simulink library "libbha_control_actuator"  (R2013b)
settings: Solver=FixedStepDiscrete  StartTime=0.0  StopTime=Inf  FixedStep=0.004  RelTol=1e-3
PostLoadFcn:
  | , if any(exist('dsrtsu_mdlpostloadfcn', 'file') == [2, 3, 6]), try dsrtsu_mdlpostloadfcn('Execute', bdroot); catch fprintf('Error in PostLoadFcn (dsrtsu_mdlpostloadfcn) for model "%s":\n %s\n', bdroot, lasterr); end, end,
undefined symbols (not defined in the file or in its folder): CONST, dim, DiscIntNeverNeededParam, tA
libraries: libbha_kinematic_tools x18, simulink x6, libbha_control_actuator x5, libbha_kinetic_cc x5, libc_control x1, libbha_parts_bellows x1, libbha_parameters x1
settings Model: DSRTSU_INTERNAL_RTI_VER=440  DSRTSU_INTERNAL_RTI_TYPE=rti1005  DSRTSU_INTERNAL_RTIFPGA=30  Creator=Falkenhahn  LastModifiedBy=Falkenhahn

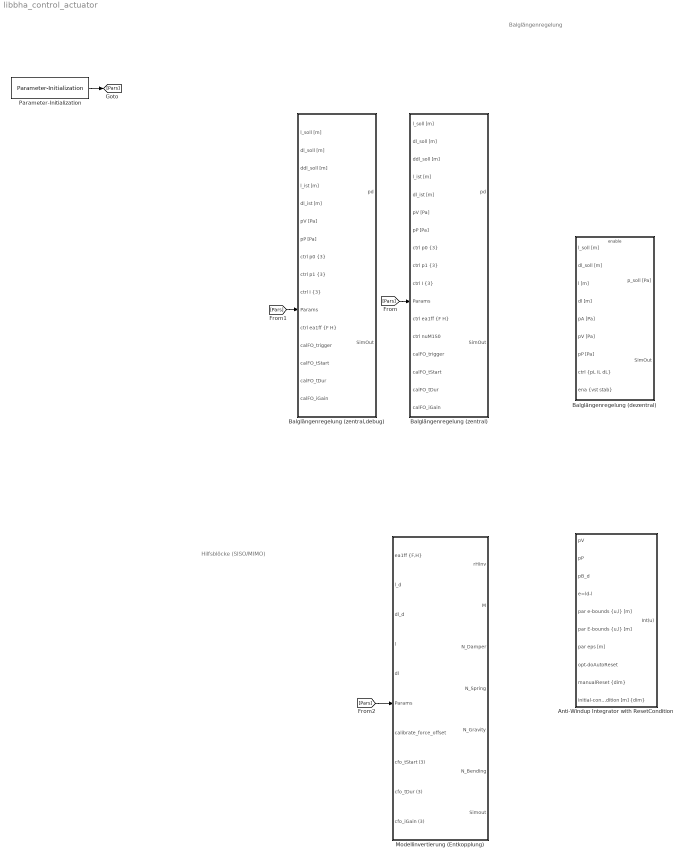
== system libbha_control_actuator ==
  note: Balglängenregelung
  note: Hilfsblöcke (SISO/MIMO)
  Anti-Windup Integrator with ResetCondition : Subsystem
      settings: AttributesFormatString=Parameter 'dim' needed\n(dimension)
  Balglängenregelung (dezentral) : Subsystem  mask{seldim=3}
      mask prompts: seldim "Dimension"
      mask init:
      | if seldim == 1
      |     dim = 1;
      | elseif seldim == 2
      |     dim = 3;
      | elseif seldim == 3
      |     dim = 6;
      | elseif seldim == 4
      |     dim = 9;
      | else
      |     dim = 1;
      | end
      settings: AttributesFormatString=%<seldim>-dimensional
      mask TypeOptions seldim: 1 | 3 | 6 | 9
  Balglängenregelung (zentral) : Subsystem
  Balglängenregelung (zentral,debug) : Subsystem
  Modellinvertierung (Entkopplung) : Subsystem
  Parameter-Initialization : libbha_parameters/Parameter-Initialization  bha_var_choice=BHA  tA=CONST.tA
      settings: AttributesFormatString=|
      | BHA-Variable: %<bha_var_choice>
      | sample time: %<tA>
  wires:
  [Pars] -> Balglängenregelung (zentral)/11(Params)
  [Pars] -> Balglängenregelung (zentral,debug)/11(Params)
  Parameter-Initialization/1 -> [Pars]
  [Pars] -> Modellinvertierung (Entkopplung)/6(Params)

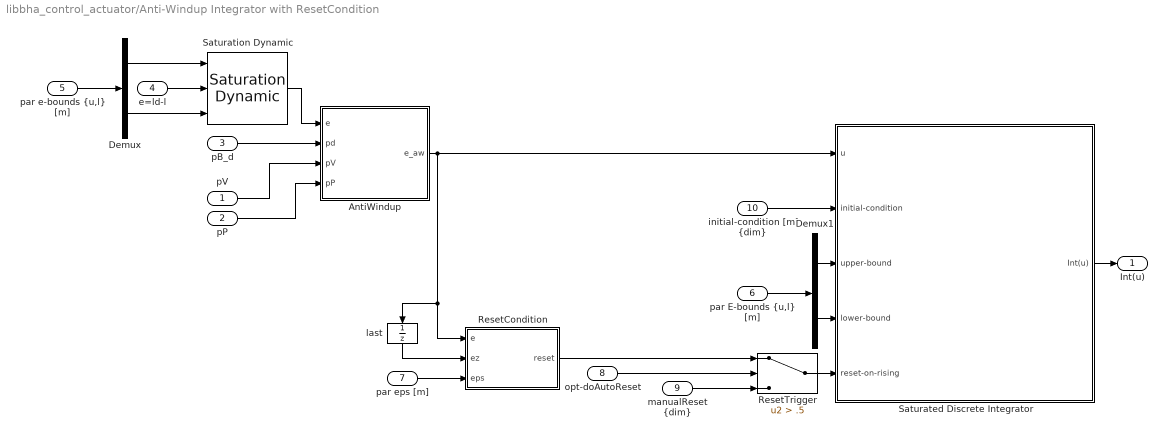
== system libbha_control_actuator/Anti-Windup Integrator with ResetCondition ==
  pV : Inport
  pP : Inport  Port=2
  pB_d : Inport  Port=3
  e=ld-l : Inport  Port=4
  "par e-bounds {u,l} [m]" : Inport  Port=5
  "par E-bounds {u,l} [m]" : Inport  Port=6
  par eps [m] : Inport  Port=7
  opt-doAutoReset : Inport  Port=8
  "manualReset {dim}" : Inport  Port=9
  "initial-condition [m] {dim}" : Inport  Port=10
  AntiWindup : MATLAB Function  TreatAsAtomicUnit=on
  Demux : Demux  Outputs=2
  Demux1 : Demux  Outputs=2
  ResetCondition : MATLAB Function  TreatAsAtomicUnit=on
  ResetTrigger : Switch  Criteria=u2 > Threshold  Threshold=.5
  Saturated Discrete Integrator : Subsystem  TreatAsAtomicUnit=on
  Saturation Dynamic : simulink/Discontinuities/Saturation Dynamic  OutMin=[]  OutMax=[]  OutDataTypeStr=Inherit: Same as second input  OutDataType=fixdt(1, 16)  OutScaling=2^-10  DoSatur=off
  last : UnitDelay  InitialCondition=zeros(dim,1)  SampleTime=-1
  Int(u) : Outport
  wires:
  pP/1 -> AntiWindup/4(pP)
  pV/1 -> AntiWindup/3(pV)
  pB_d/1 -> AntiWindup/2(pd)
  Demux/2 -> Saturation Dynamic/3
  Demux/1 -> Saturation Dynamic/1
  e=ld-l/1 -> Saturation Dynamic/2
  last/1 -> ResetCondition/2(ez)
  ResetCondition/1(reset) -> ResetTrigger/1
  Saturation Dynamic/1 -> AntiWindup/1(e)
  AntiWindup/1(e_aw) -> Saturated Discrete Integrator/1(u), ResetCondition/1(e), last/1
  Saturated Discrete Integrator/1(Int(u)) -> Int(u)/1
  ResetTrigger/1 -> Saturated Discrete Integrator/5(reset-on-rising)
  "par e-bounds {u,l} [m]"/1 -> Demux/1
  Demux1/2 -> Saturated Discrete Integrator/4(lower-bound)
  Demux1/1 -> Saturated Discrete Integrator/3(upper-bound)
  "par E-bounds {u,l} [m]"/1 -> Demux1/1
  par eps [m]/1 -> ResetCondition/3(eps)
  opt-doAutoReset/1 -> ResetTrigger/2
  "manualReset {dim}"/1 -> ResetTrigger/3
  "initial-condition [m] {dim}"/1 -> Saturated Discrete Integrator/2(initial-condition)

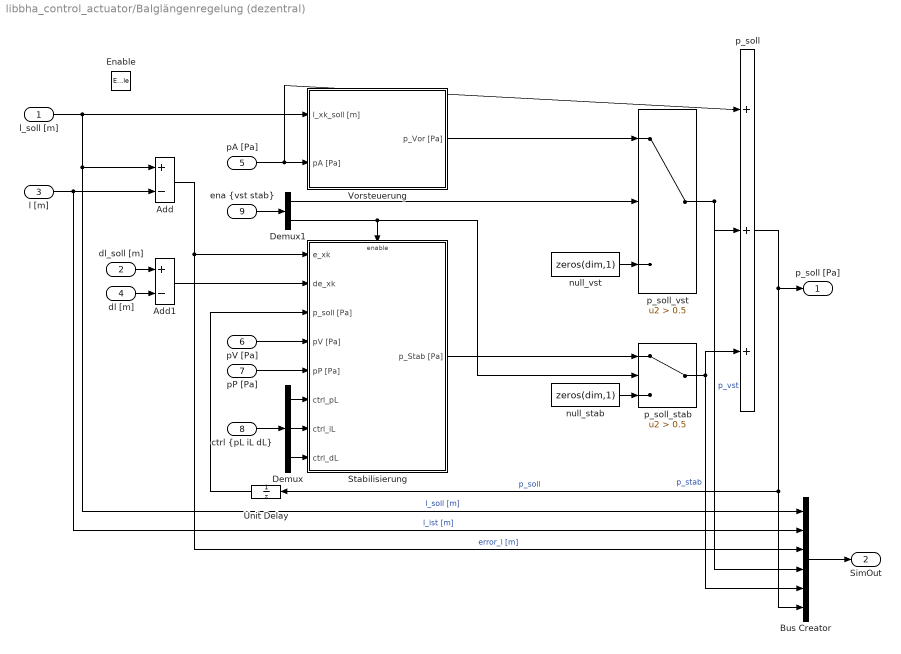
== system libbha_control_actuator/Balglängenregelung (dezentral) ==
  l_soll [m] : Inport
  dl_soll [m] : Inport  Port=2
  l [m] : Inport  Port=3
  dl [m] : Inport  Port=4
  pA [Pa] : Inport  Port=5
  pV [Pa] : Inport  Port=6
  pP [Pa] : Inport  Port=7
  "ctrl {pL iL dL}" : Inport  Port=8
  "ena {vst stab}" : Inport  Port=9
  Enable : EnablePort  StatesWhenEnabling=reset
  Add : Sum  Inputs=+-  OutDataTypeStr=Inherit: Same as first input
  Add1 : Sum  Inputs=+-  OutDataTypeStr=Inherit: Same as first input
  Bus Creator : BusCreator  Inputs=6
  Demux : Demux  Outputs=3
  Demux1 : Demux  Outputs=2
  Stabilisierung : Subsystem
  Unit Delay : UnitDelay  InitialCondition=1e5*ones(dim,1)  SampleTime=-1
  Vorsteuerung : Subsystem
  null_stab : Constant  Value=zeros(dim,1)
  null_vst : Constant  Value=zeros(dim,1)
  p_soll : Sum  Inputs=+|+||+  OutDataTypeStr=Inherit: Same as first input
  p_soll_stab : Switch  Criteria=u2 > Threshold  Threshold=0.5
  p_soll_vst : Switch  Criteria=u2 > Threshold  Threshold=0.5
  p_soll [Pa] : Outport
  SimOut : Outport  Port=2
  wires:
  Demux1/2 -> Stabilisierung/Enable, p_soll_stab/2
  "ena {vst stab}"/1 -> Demux1/1
  null_vst/1 -> p_soll_vst/3
  l [m]/1 -> Add/2, Bus Creator/2  "l_ist [m]"
  Vorsteuerung/1(p_Vor [Pa]) -> p_soll_vst/1
  pA [Pa]/1 -> Vorsteuerung/2(pA [Pa]), p_soll/1
  p_soll_stab/1 -> p_soll/3, Bus Creator/5  "p_stab"
  null_stab/1 -> p_soll_stab/3
  Demux1/1 -> p_soll_vst/2
  p_soll_vst/1 -> Bus Creator/4, p_soll/2  "p_vst"
  Stabilisierung/1(p_Stab [Pa]) -> p_soll_stab/1
  p_soll/1 -> p_soll [Pa]/1, Bus Creator/6, Unit Delay/1  "p_soll"
  l_soll [m]/1 -> Add/1, Bus Creator/1, Vorsteuerung/1(l_xk_soll [m])  "l_soll [m]"
  Unit Delay/1 -> Stabilisierung/3(p_soll [Pa])
  Bus Creator/1 -> SimOut/1
  Add/1 -> Stabilisierung/1(e_xk), Bus Creator/3  "error_l [m]"
  Demux/1 -> Stabilisierung/6(ctrl_pL)
  Demux/2 -> Stabilisierung/7(ctrl_iL)
  Demux/3 -> Stabilisierung/8(ctrl_dL)
  pV [Pa]/1 -> Stabilisierung/4(pV [Pa])
  pP [Pa]/1 -> Stabilisierung/5(pP [Pa])
  "ctrl {pL iL dL}"/1 -> Demux/1
  Add1/1 -> Stabilisierung/2(de_xk)
  dl_soll [m]/1 -> Add1/1
  dl [m]/1 -> Add1/2

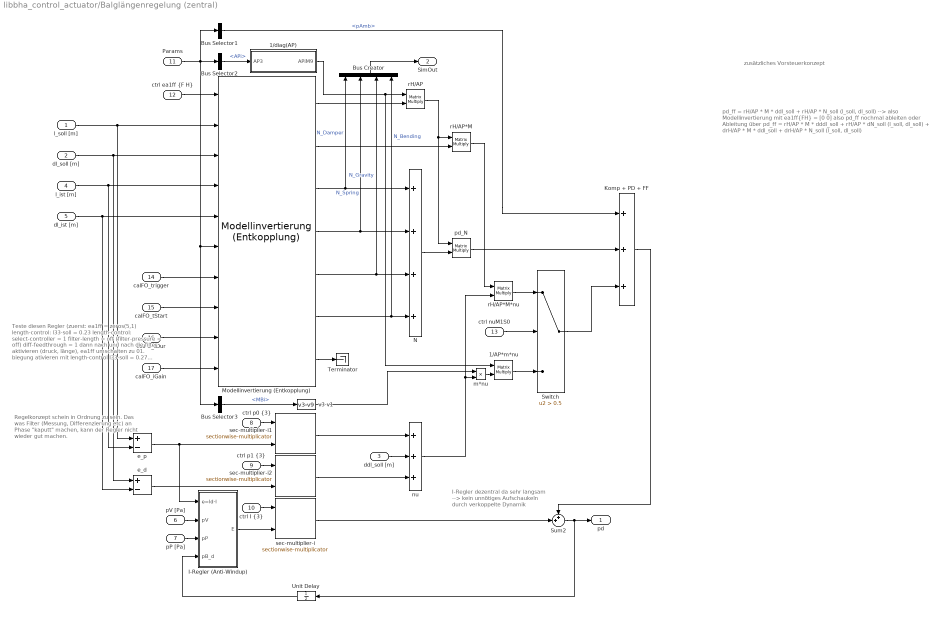
== system libbha_control_actuator/Balglängenregelung (zentral) ==
  note: I-Regler dezentral da sehr langsam
      | --> kein unnötiges Aufschaukeln
      |      durch verkoppelte Dynamik
  note: Teste diesen Regler (zuerst:
      | ea1ff = zeros(5,1)
      | length-control: l33-soll = 0.23
      | length-control: select-controller = 1
      | filter-length = off
      | (filter-pressure = off)
      | diff-feedthrough = 1
      |
      | dann nach und nach die filter aktivieren
      | (druck, länge), ea1ff umschalten zu 01.
      | biegung ativieren mit length-control l33-soll = 0.27
      | reine vorsteuerung vom dezentralen regler vergleichen
      | (achtung: link parameter verändert: ena_stab disabled!
  note: Regelkonzept schein in Ordnung zu sein.
      | Das was Filter (Messung, Differenzierung etc)
      | an Phase "kaputt" machen, kann der Regler
      | nicht wieder gut machen.
  note: zusätzliches Vorsteuerkonzept
  note: pd_ff = rH/AP * M * ddl_soll   +   rH/AP * N_soll (l_soll, dl_soll)
      |
      | --> also Modellinvertierung mit ea1ff{FH} = [0 0]
      |
      | also pd_ff nochmal ableiten oder Ableitung über
      | pd_ff = rH/AP * M * dddl_soll   +   rH/AP * dN_soll (l_soll, dl_soll)
      |          + drH/AP * M * ddl_soll   +    drH/AP * N_soll (l_soll, dl_soll)
  l_soll [m] : Inport
  dl_soll [m] : Inport  Port=2
  ddl_soll [m] : Inport  Port=3
  l_ist [m] : Inport  Port=4
  dl_ist [m] : Inport  Port=5
  pV [Pa] : Inport  Port=6
  pP [Pa] : Inport  Port=7
  "ctrl p0 {3}" : Inport  Port=8
  "ctrl p1 {3}" : Inport  Port=9
  "ctrl I {3}" : Inport  Port=10
  Params : Inport  Port=11
  "ctrl ea1ff {F H}" : Inport  Port=12
  ctrl nuM1S0 : Inport  Port=13
  calFO_trigger : Inport  Port=14
  calFO_tStart : Inport  Port=15
  calFO_tDur : Inport  Port=16
  calFO_iGain : Inport  Port=17
  1/AP*m*nu : Product  Multiplication=Matrix(*)  RndMeth=Zero
  1/diag(AP) : MATLAB Function  TreatAsAtomicUnit=on
  Bus Creator : BusCreator
  Bus Selector1 : BusSelector  OutputSignals=Pressure.pAmb
  Bus Selector2 : BusSelector  OutputSignals=Manipulator.APi
  Bus Selector3 : BusSelector  OutputSignals=Manipulator.MBi
  I-Regler (Anti-Windup) : Subsystem  mask{seldim=9}
      mask prompts: seldim "Dimension"
      mask init:
      | if seldim == 1
      |     dim = 1;
      | elseif seldim == 2
      |     dim = 3;
      | elseif seldim == 3
      |     dim = 6;
      | elseif seldim == 4
      |     dim = 9;
      | else
      |     dim = 1;
      | end
      settings: AttributesFormatString=%<seldim>-dimensional
      mask TypeOptions seldim: 1 | 3 | 6 | 9
  Komp + PD + FF : Sum  Inputs=+|+|+
  Modellinvertierung (Entkopplung) : libbha_control_actuator/Modellinvertierung (Entkopplung)
  N : Sum  Inputs=++++
  Sum2 : Sum  Inputs=++|
  Switch : Switch  Criteria=u2 > Threshold  Threshold=0.5
  Terminator : Terminator
  Unit Delay : UnitDelay  InitialCondition=1e5  SampleTime=-1
  e_d : Sum  Inputs=+-
  e_p : Sum  Inputs=+-
  m*nu : Product
  nu : Sum  Inputs=+++
  pd_N : Product  Multiplication=Matrix(*)  RndMeth=Zero
  rH/AP : Product  Multiplication=Matrix(*)  RndMeth=Zero
  rH/AP*M : Product  Multiplication=Matrix(*)  RndMeth=Zero
  rH/AP*M*nu : Product  Multiplication=Matrix(*)  RndMeth=Zero
  sec-multiplier-i : libbha_kinematic_tools/sectionwise-multiplicator
  sec-multiplier-i1 : libbha_kinematic_tools/sectionwise-multiplicator
  sec-multiplier-i2 : libbha_kinematic_tools/sectionwise-multiplicator
  v3-v1 : libbha_kinematic_tools/v3-v9
  pd : Outport
  SimOut : Outport  Port=2
  wires:
  Komp + PD + FF/1 -> Sum2/1
  calFO_tDur/1 -> Modellinvertierung (Entkopplung)/9
  calFO_iGain/1 -> Modellinvertierung (Entkopplung)/10
  calFO_tStart/1 -> Modellinvertierung (Entkopplung)/8
  Bus Selector2/1 -> 1/diag(AP)/1(AP3)  "<APi>"
  Params/1 -> Bus Selector3/1, Modellinvertierung (Entkopplung)/6, Bus Selector1/1, Bus Selector2/1
  sec-multiplier-i/1 -> Sum2/2
  Unit Delay/1 -> I-Regler (Anti-Windup)/4(pB_d)
  pP [Pa]/1 -> I-Regler (Anti-Windup)/3(pP)
  pV [Pa]/1 -> I-Regler (Anti-Windup)/2(pV)
  "ctrl I {3}"/1 -> sec-multiplier-i/1
  I-Regler (Anti-Windup)/1(E) -> sec-multiplier-i/2
  rH/AP/1 -> rH/AP*M/1, pd_N/1
  calFO_trigger/1 -> Modellinvertierung (Entkopplung)/7
  "ctrl ea1ff {F H}"/1 -> Modellinvertierung (Entkopplung)/1
  "ctrl p1 {3}"/1 -> sec-multiplier-i2/1
  "ctrl p0 {3}"/1 -> sec-multiplier-i1/1
  sec-multiplier-i2/1 -> nu/3
  sec-multiplier-i1/1 -> nu/1
  dl_ist [m]/1 -> Modellinvertierung (Entkopplung)/5, e_d/2
  l_soll [m]/1 -> Modellinvertierung (Entkopplung)/2, e_p/1
  dl_soll [m]/1 -> Modellinvertierung (Entkopplung)/3, e_d/1
  l_ist [m]/1 -> Modellinvertierung (Entkopplung)/4, e_p/2
  e_d/1 -> sec-multiplier-i2/2
  e_p/1 -> I-Regler (Anti-Windup)/1(e=ld-l), sec-multiplier-i1/2
  Modellinvertierung (Entkopplung)/7 -> Terminator/1
  rH/AP*M/1 -> rH/AP*M*nu/1
  pd_N/1 -> Komp + PD + FF/2
  Switch/1 -> Komp + PD + FF/3
  Modellinvertierung (Entkopplung)/5 -> N/3, Bus Creator/3  "N_Gravity"
  Modellinvertierung (Entkopplung)/4 -> N/2, Bus Creator/2  "N_Spring"
  Modellinvertierung (Entkopplung)/3 -> N/1, Bus Creator/1  "N_Damper"
  Modellinvertierung (Entkopplung)/6 -> N/4, Bus Creator/4  "N_Bending"
  1/diag(AP)/1(APiM9) -> 1/AP*m*nu/1, rH/AP/1
  Modellinvertierung (Entkopplung)/1 -> rH/AP/2
  Modellinvertierung (Entkopplung)/2 -> rH/AP*M/2
  Bus Creator/1 -> SimOut/1
  Sum2/1 -> pd/1, Unit Delay/1
  Bus Selector1/1 -> Komp + PD + FF/1  "<pAmb>"
  N/1 -> pd_N/2
  nu/1 -> m*nu/2, rH/AP*M*nu/2
  rH/AP*M*nu/1 -> Switch/1
  1/AP*m*nu/1 -> Switch/3
  Bus Selector3/1 -> v3-v1/1  "<MBi>"
  ddl_soll [m]/1 -> nu/2
  m*nu/1 -> 1/AP*m*nu/2
  v3-v1/1 -> m*nu/1
  ctrl nuM1S0/1 -> Switch/2

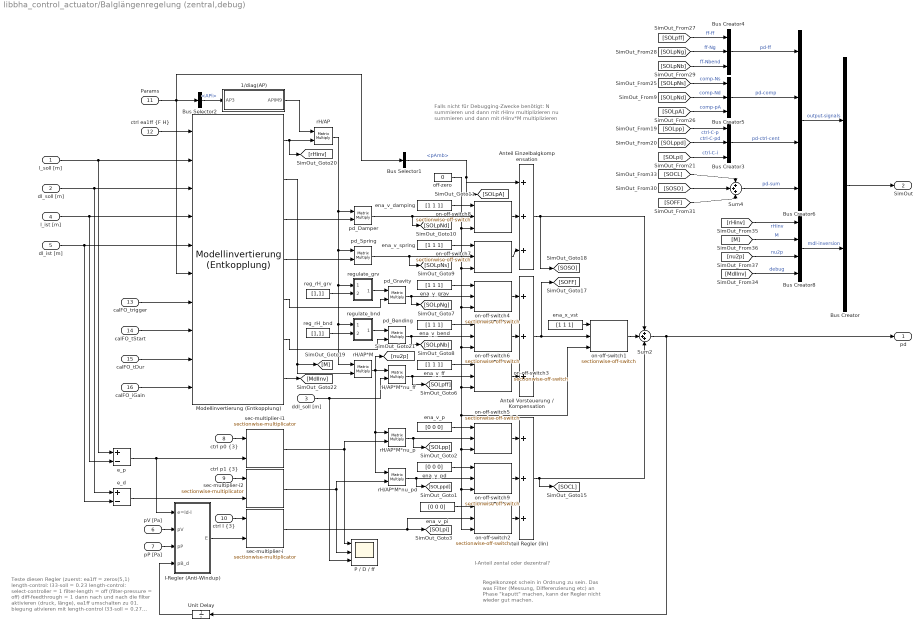
== system libbha_control_actuator/Balglängenregelung (zentral,debug) ==
  note: I-Anteil zental oder dezentral?
  note: Falls nicht für Debugging-Zwecke benötigt:
      | N summieren und dann mit rHinv multiplizieren
      | nu summieren und dann mit rHinv*M multiplizieren
  note: Regelkonzept schein in Ordnung zu sein.
      | Das was Filter (Messung, Differenzierung etc)
      | an Phase "kaputt" machen, kann der Regler
      | nicht wieder gut machen.
  note: Teste diesen Regler (zuerst:
      | ea1ff = zeros(5,1)
      | length-control: l33-soll = 0.23
      | length-control: select-controller = 1
      | filter-length = off
      | (filter-pressure = off)
      | diff-feedthrough = 1
      |
      | dann nach und nach die filter aktivieren
      | (druck, länge), ea1ff umschalten zu 01.
      | biegung ativieren mit length-control l33-soll = 0.27
      | reine vorsteuerung vom dezentralen regler vergleichen
      | (achtung: link parameter verändert: ena_stab disabled!
  l_soll [m] : Inport
  dl_soll [m] : Inport  Port=2
  ddl_soll [m] : Inport  Port=3
  l_ist [m] : Inport  Port=4
  dl_ist [m] : Inport  Port=5
  pV [Pa] : Inport  Port=6
  pP [Pa] : Inport  Port=7
  "ctrl p0 {3}" : Inport  Port=8
  "ctrl p1 {3}" : Inport  Port=9
  "ctrl I {3}" : Inport  Port=10
  Params : Inport  Port=11
  "ctrl ea1ff {F H}" : Inport  Port=12
  calFO_trigger : Inport  Port=13
  calFO_tStart : Inport  Port=14
  calFO_tDur : Inport  Port=15
  calFO_iGain : Inport  Port=16
  1/diag(AP) : MATLAB Function  TreatAsAtomicUnit=on
  Anteil Einzelbalgkompensation : Sum  Inputs=+|+|+
  Anteil Regler (lin) : Sum  Inputs=+++
  Anteil Vorsteuerung / Kompensation : Sum  Inputs=+++
  Bus Creator : BusCreator  Inputs=2
  Bus Creator3 : BusCreator  Inputs=3
  Bus Creator4 : BusCreator  Inputs=3
  Bus Creator5 : BusCreator  Inputs=3
  Bus Creator6 : BusCreator
  Bus Creator8 : BusCreator
  Bus Selector1 : BusSelector  OutputSignals=Pressure.pAmb
  Bus Selector2 : BusSelector  OutputSignals=Kinetic.APi
  I-Regler (Anti-Windup) : Subsystem  mask{seldim=9}
      mask prompts: seldim "Dimension"
      mask init:
      | if seldim == 1
      |     dim = 1;
      | elseif seldim == 2
      |     dim = 3;
      | elseif seldim == 3
      |     dim = 6;
      | elseif seldim == 4
      |     dim = 9;
      | else
      |     dim = 1;
      | end
      settings: AttributesFormatString=%<seldim>-dimensional
      mask TypeOptions seldim: 1 | 3 | 6 | 9
  Modellinvertierung (Entkopplung) : libbha_control_actuator/Modellinvertierung (Entkopplung)
  P / D / ff : Scope  NumInputPorts=3
      settings: TimeRange=10  YMin=-0.075~-0.035~-0.1  YMax=0.075~0.035~0.1
  Sum2 : Sum  Inputs=+++
  Sum4 : Sum  Inputs=+++
  Unit Delay : UnitDelay  InitialCondition=1e5  SampleTime=-1
  e_d : Sum  Inputs=+-
  e_p : Sum  Inputs=+-
  ena_v_bend : Constant  Value=[1 1 1]
  ena_v_damping : Constant  Value=[1 1 1]
  ena_v_ff : Constant  Value=[1 1 1]
  ena_v_grav : Constant  Value=[1 1 1]
  ena_v_p : Constant  Value=[0 0 0]
  ena_v_pd : Constant  Value=[0 0 0]
  ena_v_pi : Constant  Value=[0 0 0]
  ena_v_spring : Constant  Value=[1 1 1]
  ena_x_vst : Constant  Value=[1 1 1]
  off-zero : Constant  Value=0  VectorParams1D=off
  on-off-switch{1..9} (9 alike) : libbha_kinematic_tools/sectionwise-off-switch
  pd_Bending : Product  Multiplication=Matrix(*)  RndMeth=Zero
  pd_Damper : Product  Multiplication=Matrix(*)  RndMeth=Zero
  pd_Gravity : Product  Multiplication=Matrix(*)  RndMeth=Zero
  pd_Spring : Product  Multiplication=Matrix(*)  RndMeth=Zero
  rH/AP : Product  Multiplication=Matrix(*)  RndMeth=Zero
  rH/AP*M : Product  Multiplication=Matrix(*)  RndMeth=Zero
  rH/AP*M*nu_ff : Product  Multiplication=Matrix(*)  RndMeth=Zero
  rH/AP*M*nu_p : Product  Multiplication=Matrix(*)  RndMeth=Zero
  rH/AP*M*nu_pd : Product  Multiplication=Matrix(*)  RndMeth=Zero
  reg_rH_bnd : Constant  Value=[1,1]
  reg_rH_grv : Constant  Value=[1,1]
  regulate_bnd : MATLAB Function  TreatAsAtomicUnit=on
  regulate_grv : MATLAB Function  TreatAsAtomicUnit=on
  sec-multiplier-i : libbha_kinematic_tools/sectionwise-multiplicator
  sec-multiplier-i1 : libbha_kinematic_tools/sectionwise-multiplicator
  sec-multiplier-i2 : libbha_kinematic_tools/sectionwise-multiplicator
  pd : Outport
  SimOut : Outport  Port=2
  wires:
  ena_v_grav/1 -> on-off-switch4/1
  ena_v_ff/1 -> on-off-switch3/1
  ena_x_vst/1 -> on-off-switch1/1
  Anteil Vorsteuerung / Kompensation/1 -> [SOFF], on-off-switch1/2
  Bus Selector1/1 -> [SOLpA], Anteil Einzelbalgkompensation/1  "<pAmb>"
  Sum2/1 -> pd/1, Unit Delay/1
  Bus Creator/1 -> SimOut/1
  [SOLppd] -> Bus Creator3/2  "ctrl-C-pd"
  [SOLpi] -> Bus Creator3/3  "ctrl-C-i"
  [SOLpp] -> Bus Creator3/1  "ctrl-C-p"
  [SOLpNg] -> Bus Creator4/2  "ff-Ng"
  [SOLpff] -> Bus Creator4/1  "ff-ff"
  [SOLpNb] -> Bus Creator4/3  "ff-Nbend"
  [SOLpNs] -> Bus Creator5/1  "comp-Ns"
  [SOLpA] -> Bus Creator5/3  "comp-pA"
  Bus Creator4/1 -> Bus Creator6/1  "pd-ff"
  Bus Creator5/1 -> Bus Creator6/2  "pd-comp"
  Bus Creator3/1 -> Bus Creator6/3  "pd-ctrl-cent"
  Bus Creator6/1 -> Bus Creator/1  "output-signals"
  [SOSO] -> Sum4/2
  [SOFF] -> Sum4/3
  Sum4/1 -> Bus Creator6/4  "pd-sum"
  Modellinvertierung (Entkopplung)/2 -> rH/AP*M/2, [M]
  Modellinvertierung (Entkopplung)/1 -> rH/AP/2, [rHinv]
  1/diag(AP)/1(APiM9) -> rH/AP/1
  pd_Gravity/1 -> [SOLpNg], on-off-switch4/2
  ena_v_bend/1 -> on-off-switch6/1
  pd_Bending/1 -> [SOLpNb], on-off-switch6/2
  ena_v_spring/1 -> on-off-switch7/1
  pd_Spring/1 -> [SOLpNs], on-off-switch7/2
  ena_v_damping/1 -> on-off-switch8/1
  pd_Damper/1 -> [SOLpNd], on-off-switch8/2
  Modellinvertierung (Entkopplung)/6 -> pd_Bending/2
  Modellinvertierung (Entkopplung)/3 -> pd_Damper/2
  Modellinvertierung (Entkopplung)/4 -> pd_Spring/2
  Modellinvertierung (Entkopplung)/5 -> pd_Gravity/2
  on-off-switch7/1 -> Anteil Einzelbalgkompensation/3
  on-off-switch8/1 -> Anteil Einzelbalgkompensation/2
  on-off-switch6/1 -> Anteil Vorsteuerung / Kompensation/2
  on-off-switch4/1 -> Anteil Vorsteuerung / Kompensation/1
  on-off-switch3/1 -> Anteil Vorsteuerung / Kompensation/3
  off-zero/1 -> on-off-switch5/3, on-off-switch9/3, on-off-switch2/3, on-off-switch1/3, on-off-switch3/3, on-off-switch6/3, on-off-switch4/3, on-off-switch7/3, on-off-switch8/3
  rH/AP*M*nu_ff/1 -> [SOLpff], on-off-switch3/2
  rH/AP*M/1 -> [nu2p], rH/AP*M*nu_ff/1, rH/AP*M*nu_pd/1, rH/AP*M*nu_p/1
  Modellinvertierung (Entkopplung)/7 -> [MdlInv]
  [SOLpNd] -> Bus Creator5/2  "comp-Nd"
  Bus Creator8/1 -> Bus Creator/2  "mdl-inversion"
  [MdlInv] -> Bus Creator8/4  "debug"
  [rHinv] -> Bus Creator8/1  "rHinv"
  [M] -> Bus Creator8/2  "M"
  [nu2p] -> Bus Creator8/3  "nu2p"
  e_p/1 -> sec-multiplier-i1/2, I-Regler (Anti-Windup)/1(e=ld-l)
  e_d/1 -> sec-multiplier-i2/2
  l_ist [m]/1 -> e_p/2, Modellinvertierung (Entkopplung)/4
  dl_soll [m]/1 -> e_d/1, Modellinvertierung (Entkopplung)/3
  l_soll [m]/1 -> e_p/1, Modellinvertierung (Entkopplung)/2
  dl_ist [m]/1 -> e_d/2, Modellinvertierung (Entkopplung)/5
  sec-multiplier-i1/1 -> rH/AP*M*nu_p/2, P / D / ff/1
  sec-multiplier-i2/1 -> rH/AP*M*nu_pd/2, P / D / ff/2
  "ctrl p0 {3}"/1 -> sec-multiplier-i1/1
  "ctrl p1 {3}"/1 -> sec-multiplier-i2/1
  ddl_soll [m]/1 -> P / D / ff/3, rH/AP*M*nu_ff/2
  "ctrl ea1ff {F H}"/1 -> Modellinvertierung (Entkopplung)/1
  calFO_trigger/1 -> Modellinvertierung (Entkopplung)/7
  on-off-switch9/1 -> Anteil Regler (lin)/2
  on-off-switch5/1 -> Anteil Regler (lin)/1
  rH/AP*M*nu_p/1 -> on-off-switch5/2, [SOLpp]
  rH/AP*M*nu_pd/1 -> on-off-switch9/2, [SOLppd]
  ena_v_pd/1 -> on-off-switch9/1
  ena_v_p/1 -> on-off-switch5/1
  Anteil Regler (lin)/1 -> [SOCL], Sum2/3
  [SOCL] -> Sum4/1
  reg_rH_grv/1 -> regulate_grv/2(f_ud)
  regulate_grv/1(out) -> pd_Gravity/1
  rH/AP/1 -> rH/AP*M/1, regulate_bnd/1(rH), regulate_grv/1(rH), pd_Spring/1, pd_Damper/1
  regulate_bnd/1(out) -> pd_Bending/1
  reg_rH_bnd/1 -> regulate_bnd/2(f_ud)
  I-Regler (Anti-Windup)/1(E) -> sec-multiplier-i/2
  "ctrl I {3}"/1 -> sec-multiplier-i/1
  pV [Pa]/1 -> I-Regler (Anti-Windup)/2(pV)
  pP [Pa]/1 -> I-Regler (Anti-Windup)/3(pP)
  Unit Delay/1 -> I-Regler (Anti-Windup)/4(pB_d)
  sec-multiplier-i/1 -> on-off-switch2/2, [SOLpi]
  ena_v_pi/1 -> on-off-switch2/1
  on-off-switch2/1 -> Anteil Regler (lin)/3
  Params/1 -> Bus Selector2/1, Bus Selector1/1, Modellinvertierung (Entkopplung)/6
  Bus Selector2/1 -> 1/diag(AP)/1(AP3)  "<APi>"
  calFO_tStart/1 -> Modellinvertierung (Entkopplung)/8
  calFO_iGain/1 -> Modellinvertierung (Entkopplung)/10
  calFO_tDur/1 -> Modellinvertierung (Entkopplung)/9
  on-off-switch1/1 -> Sum2/2
  Anteil Einzelbalgkompensation/1 -> [SOSO], Sum2/1

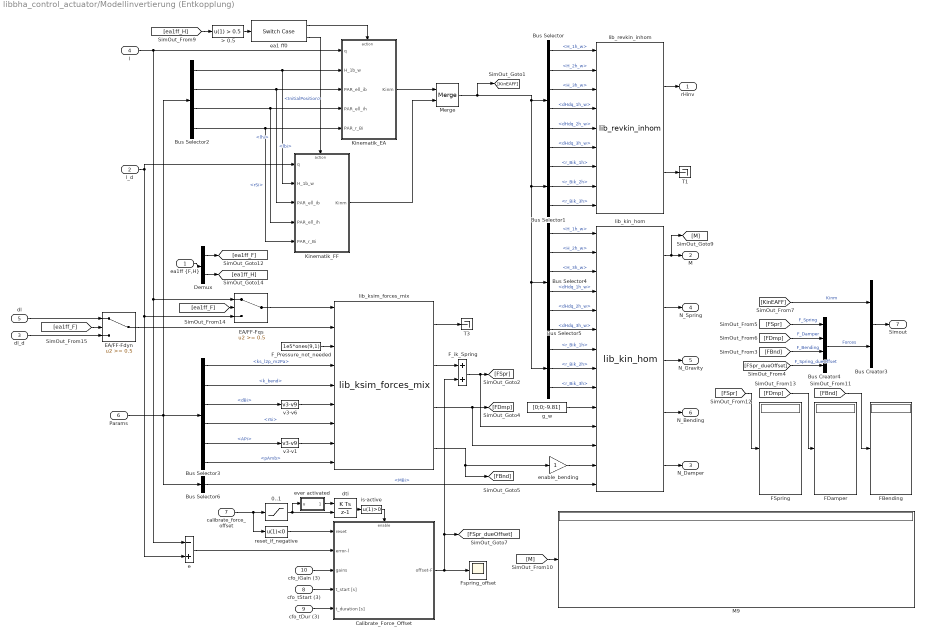
== system libbha_control_actuator/Modellinvertierung (Entkopplung) ==
  "ea1ff {F,H}" : Inport
  l_d : Inport  Port=2
  dl_d : Inport  Port=3
  l : Inport  Port=4
  dl : Inport  Port=5
  Params : Inport  Port=6
  calibrate_force_offset : Inport  Port=7
  cfo_tStart (3) : Inport  Port=8
  cfo_tDur (3) : Inport  Port=9
  cfo_iGain (3) : Inport  Port=10
  0..1 : Saturate  UpperLimit=1.0  LowerLimit=0.0
  > 0.5 : Fcn  Expr=u(1) > 0.5
  Bus Creator3 : BusCreator  Inputs=2
  Bus Creator4 : BusCreator
  Bus Selector : BusSelector  OutputSignals=H_1h_w,H_2h_w,H_3h_w,dHdq_1h_w,dHdq_2h_w,dHdq_3h_w
  Bus Selector1 : BusSelector  OutputSignals=r_Bik_1h,r_Bik_2h,r_Bik_3h
  Bus Selector2 : BusSelector  OutputSignals=Configuration.InitialPosition,Manipulator.lbi,Manipulator.lhi,Manipulator.rSi
  Bus Selector3 : BusSelector  OutputSignals=Manipulator.ks_l2p_m2Pa,Manipulator.k_bend,Manipulator.dBi,Manipulator.rSi,Manipulator.APi,Pressure.pAmb
  Bus Selector4 : BusSelector  OutputSignals=H_1h_w,H_2h_w,H_3h_w,dHdq_1h_w,dHdq_2h_w,dHdq_3h_w
  Bus Selector5 : BusSelector  OutputSignals=r_Bik_1h,r_Bik_2h,r_Bik_3h
  Bus Selector6 : BusSelector  OutputSignals=Manipulator.MBi
  Calibrate_Force_Offset : Subsystem
  Demux : Demux  Outputs=2
  EA/FF-Fdyn : Switch  Threshold=0.5
  EA/FF-Fqs : Switch  Threshold=0.5
  FBending : Display
  FDamper : Display
  FSpring : Display
  F_Pressure_not_needed : Constant  Value=1e5*ones(9,1)
  F_ik_Spring : Sum
  Fspring_offset : Scope
      settings: YMin=-35  YMax=0  SaveName=ScopeData11
  Kinematik_EA : Subsystem
      settings: AttributesFormatString=atomic unit: %<TreatAsAtomicUnit>
  Kinematik_FF : Subsystem
      settings: AttributesFormatString=atomic unit: %<TreatAsAtomicUnit>
  M9 : Display
  Merge : Merge
      settings: AttributesFormatString=|
      | schnellerer Code mit
      | switch/case statt
      | doppelte Berechnung
      | mit Schalter
  T1 : Terminator
  T3 : Terminator
  dti : DiscreteIntegrator  ExternalReset=rising  InitialCondition=-2*tA  SampleTime=tA  ICPrevOutput=DiscIntNeverNeededParam  ICPrevScaledInput=DiscIntNeverNeededParam
  e : Sum  Inputs=-+
  ea1 ff0 : SwitchCase
  enable_bending : Gain
  ever activated : Subsystem
  g_w : Constant  Value=[0;0;-9.81]  VectorParams1D=off
  is-active : Fcn  Expr=u(1)>0
  lib_kin_hom : libbha_kinetic_cc/lib_kin_hom
  lib_ksim_forces_mix : libbha_kinetic_cc/lib_ksim_forces_mix
  lib_revkin_inhom : libbha_kinetic_cc/lib_revkin_inhom
  reset_if_negative : Fcn  Expr=u(1)<0
  v3-v1 : libbha_kinematic_tools/v3-v9
  v3-v6 : libbha_kinematic_tools/v3-v9
  rHinv : Outport
  M : Outport  Port=2
  N_Damper : Outport  Port=3
  N_Spring : Outport  Port=4
  N_Gravity : Outport  Port=5
  N_Bending : Outport  Port=6
  Simout : Outport  Port=7
  wires:
  Params/1 -> Bus Selector6/1, Bus Selector2/1, Bus Selector3/1
  lib_kin_hom/1 -> M/1, [M]
  calibrate_force_offset/1 -> 0..1/1, reset_if_negative/1
  reset_if_negative/1 -> Calibrate_Force_Offset/1(reset)
  [FSpr_dueOffset] -> Bus Creator4/4  "F_Spring_dueOffset"
  cfo_tStart (3)/1 -> Calibrate_Force_Offset/4(t_start [s])
  cfo_tDur (3)/1 -> Calibrate_Force_Offset/5(t_duration [s])
  cfo_iGain (3)/1 -> Calibrate_Force_Offset/3(gains)
  dti/1 -> is-active/1
  is-active/1 -> Calibrate_Force_Offset/Enable
  ever activated/1(u>0) -> dti/1
  e/1 -> Calibrate_Force_Offset/2(error-l)
  0..1/1 -> dti/2, ever activated/1(u)
  Calibrate_Force_Offset/1(offset-F) -> Fspring_offset/1, F_ik_Spring/2, [FSpr_dueOffset]
  F_ik_Spring/1 -> lib_kin_hom/11, [FSpr]
  lib_ksim_forces_mix/2 -> F_ik_Spring/1
  l_d/1 -> e/2, EA/FF-Fqs/3, Kinematik_FF/1(q)
  l/1 -> e/1, EA/FF-Fqs/1, Kinematik_EA/1(q)
  lib_ksim_forces_mix/1 -> T3/1
  F_Pressure_not_needed/1 -> lib_ksim_forces_mix/3
  Bus Selector3/3 -> v3-v6/1  "<dBi>"
  [ea1ff_H] -> > 0.5/1
  Bus Selector6/1 -> lib_kin_hom/14  "<MBi>"
  Bus Selector2/1 -> Kinematik_EA/2(H_1b_w), Kinematik_FF/2(H_1b_w)  "<InitialPosition>"
  EA/FF-Fqs/1 -> lib_ksim_forces_mix/1
  EA/FF-Fdyn/1 -> lib_ksim_forces_mix/2
  Bus Selector3/5 -> v3-v1/1  "<APi>"
  Bus Selector3/6 -> lib_ksim_forces_mix/9  "<pAmb>"
  [ea1ff_F] -> EA/FF-Fqs/2
  [ea1ff_F] -> EA/FF-Fdyn/2
  dl_d/1 -> EA/FF-Fdyn/3
  dl/1 -> EA/FF-Fdyn/1
  lib_revkin_inhom/1 -> rHinv/1
  [FDmp] -> Bus Creator4/2  "F_Damper"
  [FBnd] -> Bus Creator4/3  "F_Bending"
  [FSpr] -> Bus Creator4/1  "F_Spring"
  [KinEAFF] -> Bus Creator3/1  "Kinm"
  Bus Creator4/1 -> Bus Creator3/2  "Forces"
  Bus Creator3/1 -> Simout/1
  [M] -> M9/1
  [FSpr] -> FSpring/1
  [FDmp] -> FDamper/1
  [FBnd] -> FBending/1
  lib_ksim_forces_mix/3 -> lib_kin_hom/12, [FDmp]
  lib_ksim_forces_mix/4 -> enable_bending/1, [FBnd]
  Bus Selector2/2 -> Kinematik_EA/3(PAR_ell_ib), Kinematik_FF/3(PAR_ell_ib)  "<lbi>"
  Bus Selector2/3 -> Kinematik_EA/4(PAR_ell_ih), Kinematik_FF/4(PAR_ell_ih)  "<lhi>"
  Bus Selector2/4 -> Kinematik_EA/5(PAR_r_Bi), Kinematik_FF/5(PAR_r_Bi)  "<rSi>"
  "ea1ff {F,H}"/1 -> Demux/1
  Demux/1 -> [ea1ff_F]
  Demux/2 -> [ea1ff_H]
  Bus Selector/1 -> lib_revkin_inhom/1  "<H_1h_w>"
  Bus Selector/6 -> lib_revkin_inhom/6  "<dHdq_3h_w>"
  Bus Selector/4 -> lib_revkin_inhom/4  "<dHdq_1h_w>"
  Bus Selector/5 -> lib_revkin_inhom/5  "<dHdq_2h_w>"
  Bus Selector/2 -> lib_revkin_inhom/2  "<H_2h_w>"
  Bus Selector/3 -> lib_revkin_inhom/3  "<H_3h_w>"
  Bus Selector1/2 -> lib_revkin_inhom/8  "<r_Bik_2h>"
  Bus Selector1/1 -> lib_revkin_inhom/7  "<r_Bik_1h>"
  Bus Selector1/3 -> lib_revkin_inhom/9  "<r_Bik_3h>"
  lib_revkin_inhom/2 -> T1/1
  Merge/1 -> Bus Selector1/1, Bus Selector4/1, Bus Selector5/1, Bus Selector/1, [KinEAFF]
  Bus Selector4/1 -> lib_kin_hom/1  "<H_1h_w>"
  Bus Selector4/6 -> lib_kin_hom/6  "<dHdq_3h_w>"
  Bus Selector4/4 -> lib_kin_hom/4  "<dHdq_1h_w>"
  Bus Selector4/5 -> lib_kin_hom/5  "<dHdq_2h_w>"
  Bus Selector4/2 -> lib_kin_hom/2  "<H_2h_w>"
  Bus Selector4/3 -> lib_kin_hom/3  "<H_3h_w>"
  Bus Selector5/2 -> lib_kin_hom/8  "<r_Bik_2h>"
  Bus Selector5/1 -> lib_kin_hom/7  "<r_Bik_1h>"
  Kinematik_FF/1(Kinm) -> Merge/2
  Bus Selector5/3 -> lib_kin_hom/9  "<r_Bik_3h>"
  g_w/1 -> lib_kin_hom/10
  lib_kin_hom/2 -> N_Spring/1
  lib_kin_hom/3 -> N_Gravity/1
  lib_kin_hom/4 -> N_Bending/1
  lib_kin_hom/5 -> N_Damper/1
  Bus Selector3/4 -> lib_ksim_forces_mix/7  "<rSi>"
  v3-v6/1 -> lib_ksim_forces_mix/6
  v3-v1/1 -> lib_ksim_forces_mix/8
  > 0.5/1 -> ea1 ff0/1
  ea1 ff0/2 -> Kinematik_FF/Action
  ea1 ff0/1 -> Kinematik_EA/Action
  Kinematik_EA/1(Kinm) -> Merge/1
  Bus Selector3/1 -> lib_ksim_forces_mix/4  "<ks_l2p_m2Pa>"
  Bus Selector3/2 -> lib_ksim_forces_mix/5  "<k_bend>"
  enable_bending/1 -> lib_kin_hom/13

== system libbha_control_actuator/Anti-Windup Integrator with ResetCondition/Saturated Discrete Integrator ==
  u : Inport  Partition=on  PartitionDimension=1  PartitionWidth=1
  initial-condition : Inport  Port=2  Partition=on  PartitionDimension=1  PartitionWidth=1
  upper-bound : Inport  Port=3  Partition=off
  lower-bound : Inport  Port=4  Partition=off
  reset-on-rising : Inport  Port=5  Partition=on  PartitionDimension=1  PartitionWidth=1
  For Each : ForEach  DisableCoverage=on  IndexMode=One-based
  Saturated Discrete Integrator : libc_control/Saturated Discrete Integrator
  Int(u) : Outport  ConcatenationDimension=1
  wires:
  Saturated Discrete Integrator/1 -> Int(u)/1
  u/1 -> Saturated Discrete Integrator/1
  initial-condition/1 -> Saturated Discrete Integrator/2
  reset-on-rising/1 -> Saturated Discrete Integrator/5
  upper-bound/1 -> Saturated Discrete Integrator/3
  lower-bound/1 -> Saturated Discrete Integrator/4

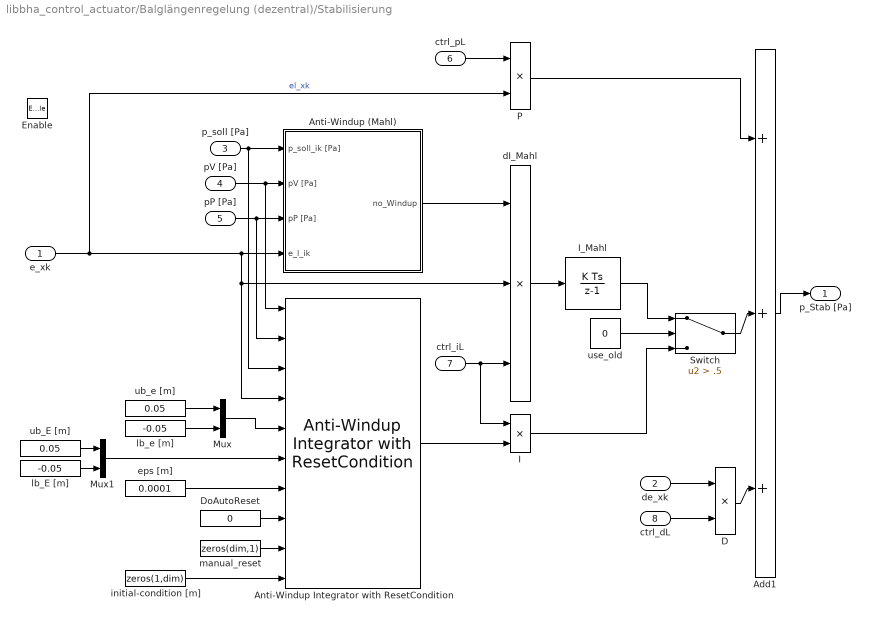
== system libbha_control_actuator/Balglängenregelung (dezentral)/Stabilisierung ==
  e_xk : Inport
  de_xk : Inport  Port=2
  p_soll [Pa] : Inport  Port=3
  pV [Pa] : Inport  Port=4
  pP [Pa] : Inport  Port=5
  ctrl_pL : Inport  Port=6
  ctrl_iL : Inport  Port=7
  ctrl_dL : Inport  Port=8
  Enable : EnablePort  StatesWhenEnabling=reset
  Add1 : Sum  Inputs=+||+|+  OutDataTypeStr=Inherit: Same as first input
  Anti-Windup (Mahl) : Subsystem
  Anti-Windup Integrator with ResetCondition : libbha_control_actuator/Anti-Windup Integrator with ResetCondition
      settings: AttributesFormatString=Parameter 'dim' needed\n(dimension)
  D : Product  RndMeth=Zero  OutDataTypeStr=Inherit: Same as first input
  DoAutoReset : Constant  Value=0
  I : Product  RndMeth=Zero  OutDataTypeStr=Inherit: Same as first input
  I_Mahl : DiscreteIntegrator  SampleTime=-1  LimitOutput=on  UpperSaturationLimit=0.5e5  LowerSaturationLimit=-0.5e5  ICPrevOutput=DiscIntNeverNeededParam  ICPrevScaledInput=DiscIntNeverNeededParam
  Mux : Mux  Inputs=2
  Mux1 : Mux  Inputs=2
  P : Product  RndMeth=Zero  OutDataTypeStr=Inherit: Same as first input
  Switch : Switch  Criteria=u2 > Threshold  Threshold=.5
  dI_Mahl : Product  Inputs=3  RndMeth=Zero  OutDataTypeStr=Inherit: Same as first input
  eps [m] : Constant  Value=0.0001
  initial-condition [m] : Constant  Value=zeros(1,dim)
  lb_E [m] : Constant  Value=-0.05
  lb_e [m] : Constant  Value=-0.05
  manual_reset : Constant  Value=zeros(dim,1)
  ub_E [m] : Constant  Value=0.05
  ub_e [m] : Constant  Value=0.05
  use_old : Constant  Value=0
  p_Stab [Pa] : Outport
  wires:
  manual_reset/1 -> Anti-Windup Integrator with ResetCondition/9
  DoAutoReset/1 -> Anti-Windup Integrator with ResetCondition/8
  initial-condition [m]/1 -> Anti-Windup Integrator with ResetCondition/10
  eps [m]/1 -> Anti-Windup Integrator with ResetCondition/7
  lb_E [m]/1 -> Mux1/2
  ub_E [m]/1 -> Mux1/1
  lb_e [m]/1 -> Mux/2
  ub_e [m]/1 -> Mux/1
  Mux1/1 -> Anti-Windup Integrator with ResetCondition/6
  Mux/1 -> Anti-Windup Integrator with ResetCondition/5
  de_xk/1 -> D/1
  I_Mahl/1 -> Switch/1
  dI_Mahl/1 -> I_Mahl/1
  Add1/1 -> p_Stab [Pa]/1
  P/1 -> Add1/1
  e_xk/1 -> P/2, Anti-Windup (Mahl)/4(e_l_ik), Anti-Windup Integrator with ResetCondition/4, dI_Mahl/2  "el_xk"
  D/1 -> Add1/3
  Anti-Windup (Mahl)/1(no_Windup) -> dI_Mahl/1
  p_soll [Pa]/1 -> Anti-Windup Integrator with ResetCondition/3, Anti-Windup (Mahl)/1(p_soll_ik [Pa])
  ctrl_pL/1 -> P/1
  ctrl_iL/1 -> dI_Mahl/3, I/1
  ctrl_dL/1 -> D/2
  pV [Pa]/1 -> Anti-Windup Integrator with ResetCondition/1, Anti-Windup (Mahl)/2(pV [Pa])
  pP [Pa]/1 -> Anti-Windup Integrator with ResetCondition/2, Anti-Windup (Mahl)/3(pP [Pa])
  Switch/1 -> Add1/2
  Anti-Windup Integrator with ResetCondition/1 -> I/2
  I/1 -> Switch/3
  use_old/1 -> Switch/2

== system libbha_control_actuator/Balglängenregelung (dezentral)/Vorsteuerung ==
  l_xk_soll [m] : Inport
  pA [Pa] : Inport  Port=2
  Stationäre Federkraft : libbha_parts_bellows/Stationäre Federkraft
      settings: AttributesFormatString=|
      | Federkennlinie als Interpolation mittels
      | Polynom 3. Ordnung mit balgspezifischen
      | Parametern p0 (konst) bis p3 (kubisch)
  Steifigkeitsparameter Balg (l->b) : Constant  Value="[ -4.04e5  5.67e6  -2.28e7  3.72e7 ]"
  p_Vor [Pa] : Outport
  wires:
  Steifigkeitsparameter Balg (l->b)/1 -> Stationäre Federkraft/3
  Stationäre Federkraft/1 -> p_Vor [Pa]/1
  pA [Pa]/1 -> Stationäre Federkraft/2
  l_xk_soll [m]/1 -> Stationäre Federkraft/1

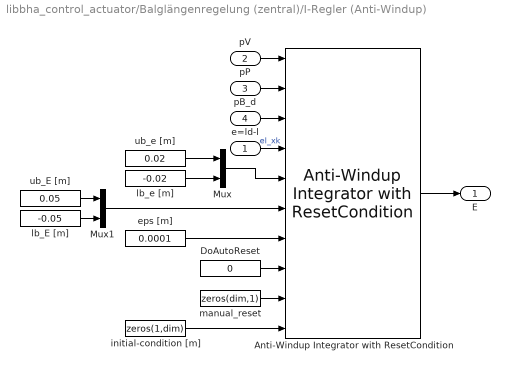
== system libbha_control_actuator/Balglängenregelung (zentral)/I-Regler (Anti-Windup) ==
  e=ld-l : Inport
  pV : Inport  Port=2
  pP : Inport  Port=3
  pB_d : Inport  Port=4
  Anti-Windup Integrator with ResetCondition : libbha_control_actuator/Anti-Windup Integrator with ResetCondition
      settings: AttributesFormatString=Parameter 'dim' needed\n(dimension)
  DoAutoReset : Constant  Value=0
  Mux : Mux  Inputs=2
  Mux1 : Mux  Inputs=2
  eps [m] : Constant  Value=0.0001
  initial-condition [m] : Constant  Value=zeros(1,dim)
  lb_E [m] : Constant  Value=-0.05
  lb_e [m] : Constant  Value=-0.02
  manual_reset : Constant  Value=zeros(dim,1)
  ub_E [m] : Constant  Value=0.05
  ub_e [m] : Constant  Value=0.02
  E : Outport
  wires:
  manual_reset/1 -> Anti-Windup Integrator with ResetCondition/9
  DoAutoReset/1 -> Anti-Windup Integrator with ResetCondition/8
  initial-condition [m]/1 -> Anti-Windup Integrator with ResetCondition/10
  eps [m]/1 -> Anti-Windup Integrator with ResetCondition/7
  lb_E [m]/1 -> Mux1/2
  ub_E [m]/1 -> Mux1/1
  lb_e [m]/1 -> Mux/2
  ub_e [m]/1 -> Mux/1
  Mux1/1 -> Anti-Windup Integrator with ResetCondition/6
  Mux/1 -> Anti-Windup Integrator with ResetCondition/5
  e=ld-l/1 -> Anti-Windup Integrator with ResetCondition/4  "el_xk"
  Anti-Windup Integrator with ResetCondition/1 -> E/1
  pB_d/1 -> Anti-Windup Integrator with ResetCondition/3
  pP/1 -> Anti-Windup Integrator with ResetCondition/2
  pV/1 -> Anti-Windup Integrator with ResetCondition/1

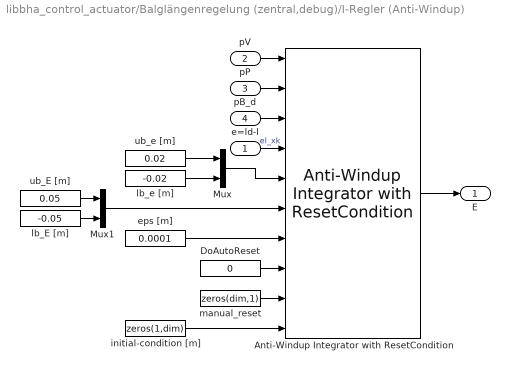
== system libbha_control_actuator/Balglängenregelung (zentral,debug)/I-Regler (Anti-Windup) ==
  e=ld-l : Inport
  pV : Inport  Port=2
  pP : Inport  Port=3
  pB_d : Inport  Port=4
  Anti-Windup Integrator with ResetCondition : libbha_control_actuator/Anti-Windup Integrator with ResetCondition
      settings: AttributesFormatString=Parameter 'dim' needed\n(dimension)
  DoAutoReset : Constant  Value=0
  Mux : Mux  Inputs=2
  Mux1 : Mux  Inputs=2
  eps [m] : Constant  Value=0.0001
  initial-condition [m] : Constant  Value=zeros(1,dim)
  lb_E [m] : Constant  Value=-0.05
  lb_e [m] : Constant  Value=-0.02
  manual_reset : Constant  Value=zeros(dim,1)
  ub_E [m] : Constant  Value=0.05
  ub_e [m] : Constant  Value=0.02
  E : Outport
  wires:
  pV/1 -> Anti-Windup Integrator with ResetCondition/1
  pP/1 -> Anti-Windup Integrator with ResetCondition/2
  pB_d/1 -> Anti-Windup Integrator with ResetCondition/3
  Anti-Windup Integrator with ResetCondition/1 -> E/1
  e=ld-l/1 -> Anti-Windup Integrator with ResetCondition/4  "el_xk"
  Mux/1 -> Anti-Windup Integrator with ResetCondition/5
  Mux1/1 -> Anti-Windup Integrator with ResetCondition/6
  ub_e [m]/1 -> Mux/1
  lb_e [m]/1 -> Mux/2
  ub_E [m]/1 -> Mux1/1
  lb_E [m]/1 -> Mux1/2
  eps [m]/1 -> Anti-Windup Integrator with ResetCondition/7
  initial-condition [m]/1 -> Anti-Windup Integrator with ResetCondition/10
  DoAutoReset/1 -> Anti-Windup Integrator with ResetCondition/8
  manual_reset/1 -> Anti-Windup Integrator with ResetCondition/9

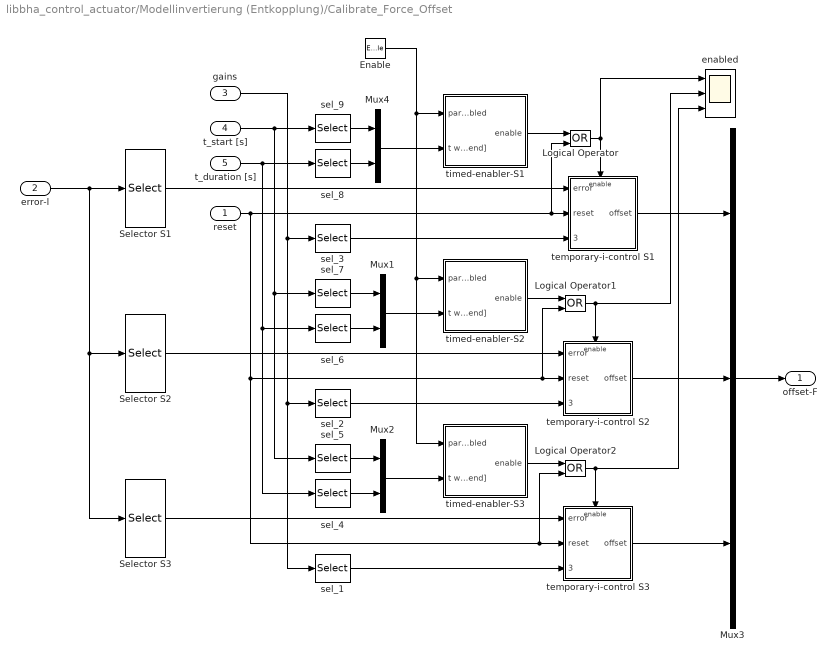
== system libbha_control_actuator/Modellinvertierung (Entkopplung)/Calibrate_Force_Offset ==
  reset : Inport
  error-l : Inport  Port=2
  gains : Inport  Port=3
  t_start [s] : Inport  Port=4
  t_duration [s] : Inport  Port=5
  Enable : EnablePort  StatesWhenEnabling=reset  ShowOutputPort=on
      settings: AttributesFormatString=%<StatesWhenEnabling> time\nwhen enabling
  Logical Operator : Logic  Operator=OR  AllPortsSameDT=off  OutDataTypeStr=boolean
  Logical Operator1 : Logic  Operator=OR  AllPortsSameDT=off  OutDataTypeStr=boolean
  Logical Operator2 : Logic  Operator=OR  AllPortsSameDT=off  OutDataTypeStr=boolean
  Mux1 : Mux  Inputs=2
  Mux2 : Mux  Inputs=2
  Mux3 : Mux  Inputs=3
  Mux4 : Mux  Inputs=2
  Selector S1 : Selector  InputPortWidth=9  IndexOptions=Index vector (dialog)  Indices=[1 2 3]  OutputSizes=1
  Selector S2 : Selector  InputPortWidth=9  IndexOptions=Index vector (dialog)  Indices=[4 5 6]  OutputSizes=1
  Selector S3 : Selector  InputPortWidth=9  IndexOptions=Index vector (dialog)  Indices=[ 7 8 9]  OutputSizes=1
  enabled : Scope  NumInputPorts=3
      settings: TimeRange=35  YMin=0~0~-2  YMax=1~1~10  SaveName=ScopeData2
  sel_1 : Selector  InputPortWidth=3  IndexOptions=Index vector (dialog)  Indices=[ 3]  OutputSizes=1
  sel_2 : Selector  InputPortWidth=3  IndexOptions=Index vector (dialog)  Indices=[ 2]  OutputSizes=1
  sel_3 : Selector  InputPortWidth=3  IndexOptions=Index vector (dialog)  Indices=[ 1]  OutputSizes=1
  sel_4 : Selector  InputPortWidth=3  IndexOptions=Index vector (dialog)  Indices=[ 3]  OutputSizes=1
  sel_5 : Selector  InputPortWidth=3  IndexOptions=Index vector (dialog)  Indices=[ 3]  OutputSizes=1
  sel_6 : Selector  InputPortWidth=3  IndexOptions=Index vector (dialog)  Indices=[ 2]  OutputSizes=1
  sel_7 : Selector  InputPortWidth=3  IndexOptions=Index vector (dialog)  Indices=[ 2]  OutputSizes=1
  sel_8 : Selector  InputPortWidth=3  IndexOptions=Index vector (dialog)  Indices=[ 1]  OutputSizes=1
  sel_9 : Selector  InputPortWidth=3  IndexOptions=Index vector (dialog)  Indices=[ 1]  OutputSizes=1
  temporary-i-control S1 : Subsystem
  temporary-i-control S2 : Subsystem
  temporary-i-control S3 : Subsystem
  timed-enabler-S1 : Subsystem
  timed-enabler-S2 : Subsystem
  timed-enabler-S3 : Subsystem
  offset-F : Outport
  wires:
  reset/1 -> Logical Operator/2, temporary-i-control S1/2(reset), Logical Operator1/2, temporary-i-control S2/2(reset), Logical Operator2/2, temporary-i-control S3/2(reset)
  t_duration [s]/1 -> sel_8/1, sel_4/1, sel_6/1
  t_start [s]/1 -> sel_9/1, sel_5/1, sel_7/1
  Mux4/1 -> timed-enabler-S1/2(t wait [start end])
  sel_8/1 -> Mux4/2
  sel_9/1 -> Mux4/1
  Mux1/1 -> timed-enabler-S2/2(t wait [start end])
  sel_7/1 -> Mux1/1
  sel_6/1 -> Mux1/2
  sel_5/1 -> Mux2/1
  sel_4/1 -> Mux2/2
  gains/1 -> sel_3/1, sel_2/1, sel_1/1
  sel_2/1 -> temporary-i-control S2/3(ctrl_gain)
  sel_3/1 -> temporary-i-control S1/3(ctrl_gain)
  sel_1/1 -> temporary-i-control S3/3(ctrl_gain)
  Selector S3/1 -> temporary-i-control S3/1(error)
  Selector S2/1 -> temporary-i-control S2/1(error)
  Selector S1/1 -> temporary-i-control S1/1(error)
  Mux3/1 -> offset-F/1
  temporary-i-control S2/1(offset) -> Mux3/2
  temporary-i-control S3/1(offset) -> Mux3/3
  temporary-i-control S1/1(offset) -> Mux3/1
  Enable/1 -> timed-enabler-S2/1(parent_enabled), timed-enabler-S3/1(parent_enabled), timed-enabler-S1/1(parent_enabled)
  Mux2/1 -> timed-enabler-S3/2(t wait [start end])
  Logical Operator2/1 -> enabled/3, temporary-i-control S3/Enable
  Logical Operator1/1 -> enabled/2, temporary-i-control S2/Enable
  Logical Operator/1 -> temporary-i-control S1/Enable, enabled/1
  error-l/1 -> Selector S2/1, Selector S3/1, Selector S1/1
  timed-enabler-S1/1(enable) -> Logical Operator/1
  timed-enabler-S3/1(enable) -> Logical Operator2/1
  timed-enabler-S2/1(enable) -> Logical Operator1/1

== system libbha_control_actuator/Modellinvertierung (Entkopplung)/Kinematik_EA ==
  q : Inport
  H_1b_w : Inport  Port=2
  PAR_ell_ib : Inport  Port=3
  PAR_ell_ih : Inport  Port=4
  PAR_r_Bi : Inport  Port=5
  Action Port : ActionPort  ActionType=case
  Bus Creator : BusCreator  Inputs=9
  Signal Conversion : SignalConversion
  lib_kinm : libbha_kinetic_cc/lib_kinm
  Kinm : Outport
  wires:
  Bus Creator/1 -> Signal Conversion/1
  PAR_ell_ib/1 -> lib_kinm/3
  PAR_ell_ih/1 -> lib_kinm/4
  q/1 -> lib_kinm/1
  H_1b_w/1 -> lib_kinm/2
  PAR_r_Bi/1 -> lib_kinm/5
  lib_kinm/9 -> Bus Creator/9  "r_Bik_3h"
  lib_kinm/2 -> Bus Creator/2  "H_2h_w"
  lib_kinm/7 -> Bus Creator/7  "r_Bik_1h"
  lib_kinm/1 -> Bus Creator/1  "H_1h_w"
  lib_kinm/8 -> Bus Creator/8  "r_Bik_2h"
  lib_kinm/4 -> Bus Creator/4  "dHdq_1h_w"
  lib_kinm/6 -> Bus Creator/6  "dHdq_3h_w"
  lib_kinm/5 -> Bus Creator/5  "dHdq_2h_w"
  lib_kinm/3 -> Bus Creator/3  "H_3h_w"
  Signal Conversion/1 -> Kinm/1

== system libbha_control_actuator/Modellinvertierung (Entkopplung)/Kinematik_FF ==
  q : Inport
  H_1b_w : Inport  Port=2
  PAR_ell_ib : Inport  Port=3
  PAR_ell_ih : Inport  Port=4
  PAR_r_Bi : Inport  Port=5
  Action Port : ActionPort  ActionType=default
  Bus Creator : BusCreator  Inputs=9
  Signal Conversion : SignalConversion
  lib_kinm : libbha_kinetic_cc/lib_kinm
  Kinm : Outport
  wires:
  lib_kinm/3 -> Bus Creator/3  "H_3h_w"
  lib_kinm/5 -> Bus Creator/5  "dHdq_2h_w"
  lib_kinm/6 -> Bus Creator/6  "dHdq_3h_w"
  lib_kinm/4 -> Bus Creator/4  "dHdq_1h_w"
  lib_kinm/8 -> Bus Creator/8  "r_Bik_2h"
  lib_kinm/1 -> Bus Creator/1  "H_1h_w"
  lib_kinm/7 -> Bus Creator/7  "r_Bik_1h"
  lib_kinm/2 -> Bus Creator/2  "H_2h_w"
  lib_kinm/9 -> Bus Creator/9  "r_Bik_3h"
  PAR_r_Bi/1 -> lib_kinm/5
  H_1b_w/1 -> lib_kinm/2
  q/1 -> lib_kinm/1
  PAR_ell_ih/1 -> lib_kinm/4
  PAR_ell_ib/1 -> lib_kinm/3
  Bus Creator/1 -> Signal Conversion/1
  Signal Conversion/1 -> Kinm/1

== system libbha_control_actuator/Modellinvertierung (Entkopplung)/ever activated ==
  u : Inport
  Compare To Zero : simulink/Logic and Bit Operations/Compare To Zero  relop=>  OutDataTypeStr=boolean
  Data Type Conversion : DataTypeConversion
  speicher : DiscreteIntegrator  InitialCondition=-CONST.tA  SampleTime=-1  LimitOutput=on  LowerSaturationLimit=-CONST.tA  ICPrevOutput=DiscIntNeverNeededParam  ICPrevScaledInput=DiscIntNeverNeededParam
  u>0 : Outport
  wires:
  Data Type Conversion/1 -> u>0/1
  u/1 -> speicher/1
  speicher/1 -> Compare To Zero/1
  Compare To Zero/1 -> Data Type Conversion/1

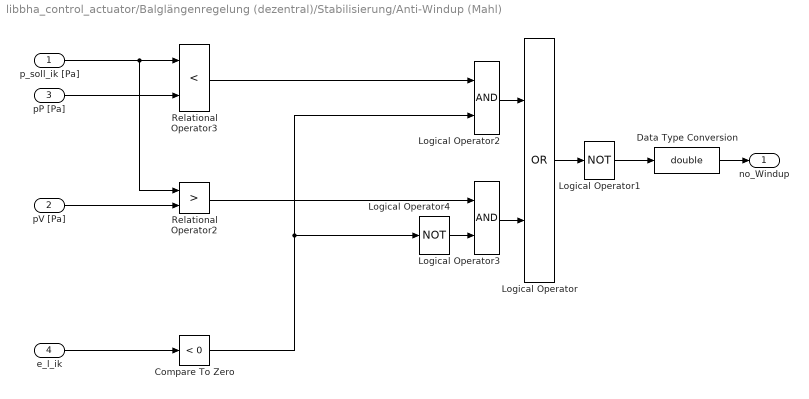
== system libbha_control_actuator/Balglängenregelung (dezentral)/Stabilisierung/Anti-Windup (Mahl) ==
  p_soll_ik [Pa] : Inport
  pV [Pa] : Inport  Port=2
  pP [Pa] : Inport  Port=3
  e_l_ik : Inport  Port=4
  Compare To Zero : simulink/Logic and Bit Operations/Compare To Zero  relop=<  OutDataTypeStr=uint8
  Data Type Conversion : DataTypeConversion  OutDataTypeStr=double
  Logical Operator : Logic  Operator=OR  AllPortsSameDT=off  OutDataTypeStr=boolean
  Logical Operator1 : Logic  Operator=NOT  AllPortsSameDT=off  OutDataTypeStr=boolean
  Logical Operator2 : Logic  AllPortsSameDT=off  OutDataTypeStr=boolean
  Logical Operator3 : Logic  AllPortsSameDT=off  OutDataTypeStr=boolean
  Logical Operator4 : Logic  Operator=NOT  AllPortsSameDT=off  OutDataTypeStr=boolean
  Relational Operator2 : RelationalOperator  Operator=>  OutDataTypeStr=boolean
  Relational Operator3 : RelationalOperator  Operator=<  OutDataTypeStr=boolean
  no_Windup : Outport
  wires:
  Relational Operator3/1 -> Logical Operator2/1
  Relational Operator2/1 -> Logical Operator3/1
  p_soll_ik [Pa]/1 -> Relational Operator3/1, Relational Operator2/1
  pP [Pa]/1 -> Relational Operator3/2
  Logical Operator/1 -> Logical Operator1/1
  e_l_ik/1 -> Compare To Zero/1
  Compare To Zero/1 -> Logical Operator2/2, Logical Operator4/1
  Logical Operator1/1 -> Data Type Conversion/1
  Data Type Conversion/1 -> no_Windup/1
  Logical Operator2/1 -> Logical Operator/1
  Logical Operator3/1 -> Logical Operator/2
  Logical Operator4/1 -> Logical Operator3/2
  pV [Pa]/1 -> Relational Operator2/2

== system libbha_control_actuator/Modellinvertierung (Entkopplung)/Calibrate_Force_Offset/temporary-i-control S1 ==
  error : Inport
  reset : Inport  Port=2
  ctrl_gain : Inport  Port=3
  Enable : EnablePort
      settings: AttributesFormatString=%<StatesWhenEnabling> offset\nwhen enabling
  Product : Product  RndMeth=Zero
  dti : DiscreteIntegrator  ExternalReset=level  SampleTime=-1  ICPrevOutput=DiscIntNeverNeededParam  ICPrevScaledInput=DiscIntNeverNeededParam
  offset : Outport
  wires:
  reset/1 -> dti/2
  dti/1 -> offset/1
  Product/1 -> dti/1
  error/1 -> Product/1
  ctrl_gain/1 -> Product/2

== system libbha_control_actuator/Modellinvertierung (Entkopplung)/Calibrate_Force_Offset/temporary-i-control S2 ==
  error : Inport
  reset : Inport  Port=2
  ctrl_gain : Inport  Port=3
  Enable : EnablePort
      settings: AttributesFormatString=%<StatesWhenEnabling> offset\nwhen enabling
  Product : Product  RndMeth=Zero
  dti : DiscreteIntegrator  ExternalReset=level  SampleTime=-1  ICPrevOutput=DiscIntNeverNeededParam  ICPrevScaledInput=DiscIntNeverNeededParam
  offset : Outport
  wires:
  ctrl_gain/1 -> Product/2
  error/1 -> Product/1
  Product/1 -> dti/1
  dti/1 -> offset/1
  reset/1 -> dti/2

== system libbha_control_actuator/Modellinvertierung (Entkopplung)/Calibrate_Force_Offset/temporary-i-control S3 ==
  error : Inport
  reset : Inport  Port=2
  ctrl_gain : Inport  Port=3
  Enable : EnablePort
      settings: AttributesFormatString=%<StatesWhenEnabling> offset\nwhen enabling
  Product : Product  RndMeth=Zero
  dti : DiscreteIntegrator  ExternalReset=level  SampleTime=-1  ICPrevOutput=DiscIntNeverNeededParam  ICPrevScaledInput=DiscIntNeverNeededParam
  offset : Outport
  wires:
  reset/1 -> dti/2
  dti/1 -> offset/1
  Product/1 -> dti/1
  error/1 -> Product/1
  ctrl_gain/1 -> Product/2

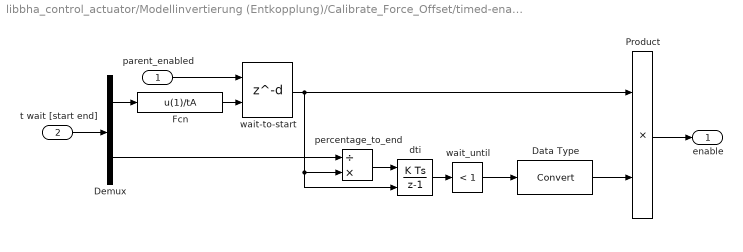
== system libbha_control_actuator/Modellinvertierung (Entkopplung)/Calibrate_Force_Offset/timed-enabler-S1 ==
  parent_enabled : Inport
  t wait [start end] : Inport  Port=2
  Data Type : DataTypeConversion
  Demux : Demux  Outputs=2
  Fcn : Fcn  Expr=u(1)/tA
  Product : Product  RndMeth=Zero
  dti : DiscreteIntegrator  ExternalReset=rising  SampleTime=-1  ICPrevOutput=DiscIntNeverNeededParam  ICPrevScaledInput=DiscIntNeverNeededParam
  percentage_to_end : Product  Inputs=/*  RndMeth=Zero
  wait-to-start : Delay  DelayLengthSource=Input port  DelayLength=1/CONST.tA  DelayLengthUpperLimit=10/tA  SampleTime=tA
      settings: InputPortMap=u0,p1
  wait_until : simulink/Logic and Bit Operations/Compare To Constant  relop=<  const=1  OutDataTypeStr=boolean
  enable : Outport
  wires:
  parent_enabled/1 -> wait-to-start/1
  Fcn/1 -> wait-to-start/2
  Demux/1 -> Fcn/1
  dti/1 -> wait_until/1
  wait_until/1 -> Data Type/1
  percentage_to_end/1 -> dti/1
  Demux/2 -> percentage_to_end/1
  wait-to-start/1 -> dti/2, percentage_to_end/2, Product/1
  Product/1 -> enable/1
  Data Type/1 -> Product/2
  t wait [start end]/1 -> Demux/1

== system libbha_control_actuator/Modellinvertierung (Entkopplung)/Calibrate_Force_Offset/timed-enabler-S2 ==
  parent_enabled : Inport
  t wait [start end] : Inport  Port=2
  Data Type : DataTypeConversion
  Demux : Demux  Outputs=2
  Fcn : Fcn  Expr=u(1)/tA
  Product : Product  RndMeth=Zero
  dti : DiscreteIntegrator  ExternalReset=rising  SampleTime=-1  ICPrevOutput=DiscIntNeverNeededParam  ICPrevScaledInput=DiscIntNeverNeededParam
  percentage_to_end : Product  Inputs=/*  RndMeth=Zero
  wait-to-start : Delay  DelayLengthSource=Input port  DelayLength=1/CONST.tA  DelayLengthUpperLimit=10/tA  SampleTime=tA
      settings: InputPortMap=u0,p1
  wait_until : simulink/Logic and Bit Operations/Compare To Constant  relop=<  const=1  OutDataTypeStr=boolean
  enable : Outport
  wires:
  t wait [start end]/1 -> Demux/1
  Data Type/1 -> Product/2
  Product/1 -> enable/1
  wait-to-start/1 -> Product/1, percentage_to_end/2, dti/2
  Demux/2 -> percentage_to_end/1
  percentage_to_end/1 -> dti/1
  wait_until/1 -> Data Type/1
  dti/1 -> wait_until/1
  Demux/1 -> Fcn/1
  Fcn/1 -> wait-to-start/2
  parent_enabled/1 -> wait-to-start/1

== system libbha_control_actuator/Modellinvertierung (Entkopplung)/Calibrate_Force_Offset/timed-enabler-S3 ==
  parent_enabled : Inport
  t wait [start end] : Inport  Port=2
  Data Type : DataTypeConversion
  Demux : Demux  Outputs=2
  Fcn : Fcn  Expr=u(1)/tA
  Product : Product  RndMeth=Zero
  dti : DiscreteIntegrator  ExternalReset=rising  SampleTime=-1  ICPrevOutput=DiscIntNeverNeededParam  ICPrevScaledInput=DiscIntNeverNeededParam
  percentage_to_end : Product  Inputs=/*  RndMeth=Zero
  wait-to-start : Delay  DelayLengthSource=Input port  DelayLength=1/CONST.tA  DelayLengthUpperLimit=10/tA  SampleTime=tA
      settings: InputPortMap=u0,p1
  wait_until : simulink/Logic and Bit Operations/Compare To Constant  relop=<  const=1  OutDataTypeStr=boolean
  enable : Outport
  wires:
  parent_enabled/1 -> wait-to-start/1
  Fcn/1 -> wait-to-start/2
  Demux/1 -> Fcn/1
  dti/1 -> wait_until/1
  wait_until/1 -> Data Type/1
  percentage_to_end/1 -> dti/1
  Demux/2 -> percentage_to_end/1
  wait-to-start/1 -> dti/2, percentage_to_end/2, Product/1
  Product/1 -> enable/1
  Data Type/1 -> Product/2
  t wait [start end]/1 -> Demux/1

== matlab function libbha_control_actuator/Anti-Windup Integrator with ResetCondition/AntiWindup ==
  data: e input; e_aw output; pd input; pV input; pP input
function e_aw = antiwindup(e, pd, pV, pP)
% Integration nur erlaubt wenn

%  1. Druckbereich eingehalten oder aus Druckbegrenzung herausgefahren wird
%       a) Druck kleiner als Versorgungsdruck (oder Strecke soll verkleinert werden)
%       b) Druck größer als Versorgungsdruck (oder Strecke soll vergrößert werden)

    e_aw = e;

    for i=1:length(e)
        %if (pd(i) < pV || e(i) < 0 ) && (pd(i) > pP || e(i) > 0)
        %    e_aw(i) = e(i);
        %else
        if (pd(i) > pV && e(i) < 0 ) || (pd(i) < pP && e(i) > 0)
            e_aw(i) = 0.0;
        end
    end

end

== matlab function libbha_control_actuator/Anti-Windup Integrator with ResetCondition/ResetCondition ==
  data: e input; reset output; ez input; eps input
function reset = reset(e, ez, eps)
% Zurücksetzten, wenn

%  1. Fehler klein (eps) oder der Fehler seit dem letzten Zeitschritt das
%     Vorzeichen gewechselt hat (zero crossing)

    reset = 0*e;

    for i=1:length(e)
        if abs(e(i)) <= eps || e(i)*ez(i) <= 0
            reset(i) = 1.0;
        %else
        %    reset = 0.0;
        end
    end

end

== matlab function libbha_control_actuator/Balglängenregelung (zentral,debug)/1//diag(AP) ==
  data: AP3 input; APiM9 output
function APiM9 = invDiagAP(AP3)
    APi3 = 1./AP3;
    APi9 = [APi3(1);APi3(1);APi3(1);APi3(2);APi3(2);APi3(2);APi3(3);APi3(3);APi3(3)];
    APiM9 = diag(APi9);
end

== matlab function libbha_control_actuator/Balglängenregelung (zentral,debug)/regulate_bnd ==
  data: rH input; out output; f_ud input
function out = reg(rH,f_ud)

out = rH;
out(1:3,4:9) = f_ud(1)*rH(1:3,4:9);
out(4:6,7:9) = f_ud(1)*rH(4:6,7:9);

out(4:6,1:3) = f_ud(2)*rH(4:6,1:3);
out(7:9,1:6) = f_ud(2)*rH(7:9,1:6);

== matlab function libbha_control_actuator/Balglängenregelung (zentral,debug)/regulate_grv ==
  data: rH input; out output; f_ud input
function out = reg(rH,f_ud)

out = rH;
out(1:3,4:9) = f_ud(1)*rH(1:3,4:9);
out(4:6,7:9) = f_ud(1)*rH(4:6,7:9);

out(4:6,1:3) = f_ud(2)*rH(4:6,1:3);
out(7:9,1:6) = f_ud(2)*rH(7:9,1:6);

== matlab function libbha_control_actuator/Balglängenregelung (zentral)/1//diag(AP) ==
  data: AP3 input; APiM9 output
function APiM9 = invDiagAP(AP3)
    APi3 = 1./AP3;
    APi9 = [APi3(1);APi3(1);APi3(1);APi3(2);APi3(2);APi3(2);APi3(3);APi3(3);APi3(3)];
    APiM9 = diag(APi9);
end
